simulink model "CoupledSystem"  (R2021b)
settings: Solver=ode1  StartTime=0.0  StopTime=10.0  FixedStep=0.001  RelTol=1e-3
settings Model: Creator=au602135  LastModifiedBy=au602135

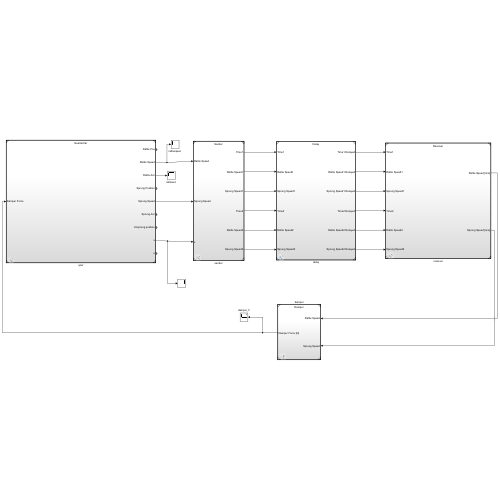
[thumbnail: Simulink's stored preview of the top-level diagram]
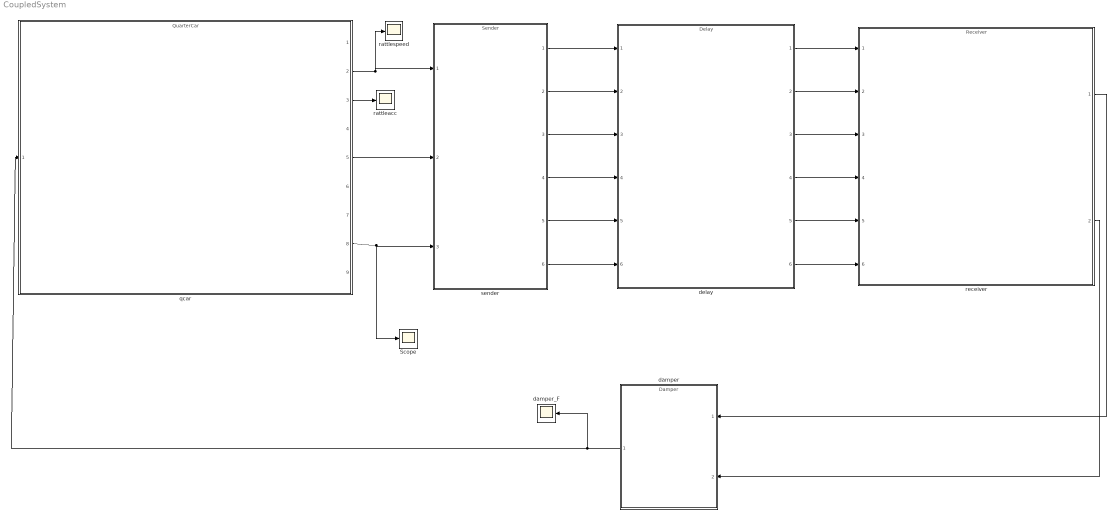
== system CoupledSystem ==
  Scope : Scope
  damper : ModelReference  ModelNameDialog=Damper.slx  SimulationMode=Normal  ModelReferenceVersion=11.2
  damper_F : Scope
  delay : ModelReference  ModelNameDialog=Delay.slx  SimulationMode=Normal  ModelReferenceVersion=11.4
  qcar : ModelReference  ModelNameDialog=QuarterCar.slx  SimulationMode=Normal  ModelReferenceVersion=11.7
  rattleacc : Scope
  rattlespeed : Scope
  receiver : ModelReference  ModelNameDialog=Receiver.slx  SimulationMode=Normal  ModelReferenceVersion=11.2
  sender : ModelReference  ModelNameDialog=Sender.slx  SimulationMode=Normal  ModelReferenceVersion=11.4
  wires:
  qcar/2 -> rattlespeed/1, sender/1
  qcar/5 -> sender/2
  qcar/8 -> Scope/1, sender/3
  sender/1 -> delay/1
  sender/2 -> delay/2
  sender/3 -> delay/3
  sender/4 -> delay/4
  sender/5 -> delay/5
  sender/6 -> delay/6
  delay/1 -> receiver/1
  delay/2 -> receiver/2
  delay/3 -> receiver/3
  delay/4 -> receiver/4
  delay/5 -> receiver/5
  delay/6 -> receiver/6
  receiver/1 -> damper/1
  receiver/2 -> damper/2
  damper/1 -> damper_F/1, qcar/1
  qcar/3 -> rattleacc/1
